simulink model "Test_Byte_Demultiplexer_1_to_8"  (Simulink 8.1)
settings: Solver=ode45  StartTime=0.0  StopTime=len  RelTol=1e-3
libraries: Byte_Demultiplexers_Lib x1, commutil2 x1
settings Model: Creator=N  LastModifiedBy=uzivatel
settings DataIOCC: LimitDataPoints=off  SignalLoggingSaveFormat=Dataset
settings OptimizationCC: ExpressionDepthLimit=128
settings DebuggingCC: UnderspecifiedInitializationDetection=Simplified  MergeDetectMultiDrivingBlocksExec=error  SolverPrmCheckMsg=none  FcnCallInpInsideContextMsg=EnableAllAsError  FrameProcessingCompatibilityMsg=error  StateNameClashWarn=none
settings HardwareCC: ProdBitPerPointer=64  ProdLargestAtomicFloat=Float  ProdIntDivRoundTo=Zero  ProdEndianess=LittleEndian  ProdHWDeviceType=Intel->x86-64 (Windows64)
settings ModelReferenceCC: PropagateSignalLabelsOutOfModel=on
settings GRTTargetCC: CodeReplacementLibrary=None  CombineOutputUpdateFcns=on  CPPClassGenCompliant=on  GRTInterface=off

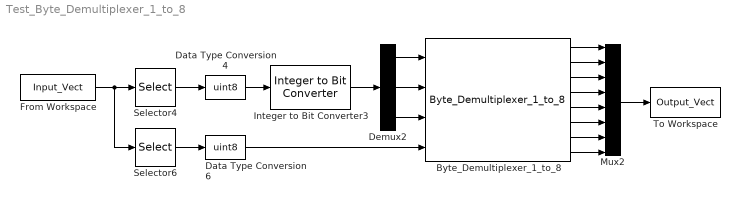
== system Test_Byte_Demultiplexer_1_to_8 ==
  Byte_Demultiplexer_1_to_8 : Byte_Demultiplexers_Lib/Byte_Demultiplexers_Lib/Byte_Demultiplexer_1_to_8
  Data Type Conversion4 : DataTypeConversion  OutDataTypeStr=uint8
  Data Type Conversion6 : DataTypeConversion  OutDataTypeStr=uint8
  Demux2 : Demux  Outputs=3
  From Workspace : FromWorkspace  VariableName=Input_Vect  SampleTime=1  Interpolate=off  OutputAfterFinalValue=Holding final value
  Integer to Bit Converter3 : commutil2/Integer to Bit Converter  nbits=3  signedInputValues=Unsigned  bitOrder=MSB first  outDtype=boolean
  Mux2 : Mux  Inputs=8
  Selector4 : Selector  IndexMode=Zero-based  InputPortWidth=2  SampleTime=1  IndexOptions=Index vector (dialog)  Indices=0  OutputSizes=1
  Selector6 : Selector  IndexMode=Zero-based  InputPortWidth=2  IndexOptions=Index vector (dialog)  Indices=1  OutputSizes=1
  To Workspace : ToWorkspace  VariableName=Output_Vect  SampleTime=1
  wires:
  Integer to Bit Converter3/1 -> Demux2/1
  Selector4/1 -> Data Type Conversion4/1
  Data Type Conversion4/1 -> Integer to Bit Converter3/1
  From Workspace/1 -> Selector6/1, Selector4/1
  Demux2/1 -> Byte_Demultiplexer_1_to_8/1
  Demux2/2 -> Byte_Demultiplexer_1_to_8/2
  Demux2/3 -> Byte_Demultiplexer_1_to_8/3
  Selector6/1 -> Data Type Conversion6/1
  Data Type Conversion6/1 -> Byte_Demultiplexer_1_to_8/4
  Mux2/1 -> To Workspace/1
  Byte_Demultiplexer_1_to_8/1 -> Mux2/1
  Byte_Demultiplexer_1_to_8/8 -> Mux2/8
  Byte_Demultiplexer_1_to_8/2 -> Mux2/2
  Byte_Demultiplexer_1_to_8/3 -> Mux2/3
  Byte_Demultiplexer_1_to_8/4 -> Mux2/4
  Byte_Demultiplexer_1_to_8/5 -> Mux2/5
  Byte_Demultiplexer_1_to_8/6 -> Mux2/6
  Byte_Demultiplexer_1_to_8/7 -> Mux2/7
